simulink model "hexapod"  (R2015a)
settings: Solver=ode23tb  StartTime=0.0  StopTime=10  FixedStep=0.001  MaxStep=0.01  RelTol=1e-4  AbsTol=1e-5
values from neighbouring files (symbols this model uses):
  bL = 18.5    [runFirst.m]    (also in runFirst2.m = 20.5)
  bWb = 12.5    [runFirst.m]    (also in runFirst2.m = 14.5)
  bWs = 10.5    [runFirst.m]    (also in runFirst2.m = 12.5)
  C = CM + CL/n^2    (= 0.0001377500155)    [runFirst.m]
  d1 = 0    [runFirst.m]    (also in runFirst2.m)
  d2 = -4.61    [runFirst.m]    (also in runFirst2.m = 0)
  J = JM + JL/n^2    (= 0.008455500031)    [runFirst.m]
  Ka = 12    [runFirst.m]
  Kb = 0.00867    [runFirst.m]
  Ke = 1    [runFirst.m]
  Km = 4.375    [runFirst.m]
  L = 0.0006    [runFirst.m]
  L1 = 3.64    [runFirst.m]    (also in runFirst2.m = 3.4)
  l1x = 15.78    [runFirst.m]
  l1y = 11.78    [runFirst.m]
  l1z = -14.9    [runFirst.m]
  L2 = 5.72    [runFirst.m]    (also in runFirst2.m = 8.7)
  l2x = 0    [runFirst.m]
  l2y = 15.48    [runFirst.m]
  l2z = -14.9    [runFirst.m]
  L3 = 12.46    [runFirst.m]    (also in runFirst2.m = 12.73)
  l3x = -15.78    [runFirst.m]
  l3y = 11.78    [runFirst.m]
  l3z = -14.9    [runFirst.m]
  l4x = 15.78    [runFirst.m]
  l4y = -11.78    [runFirst.m]
  l4z = -14.9    [runFirst.m]
  l5x = 0    [runFirst.m]
  l5y = -15.48    [runFirst.m]
  l5z = -14.9    [runFirst.m]
  l6x = -15.78    [runFirst.m]
  l6y = -11.78    [runFirst.m]
  l6z = -14.9    [runFirst.m]
  n = 254    [runFirst.m]
  R = 1.4    [runFirst.m]
  stX = 4    [runFirst.m]
  stZ = 2    [runFirst.m]
  Ts = 2    [runFirst.m]
undefined symbols (not defined in the file or in its folder): X, Y, Z
undefined symbols (not defined in the file): bH, bM, m1, m2, m3
libraries: sm_lib x108, nesl_utility x52, simulink x12, Contact_Forces_Lib x7, roblocks x2
(part 2 of 5)

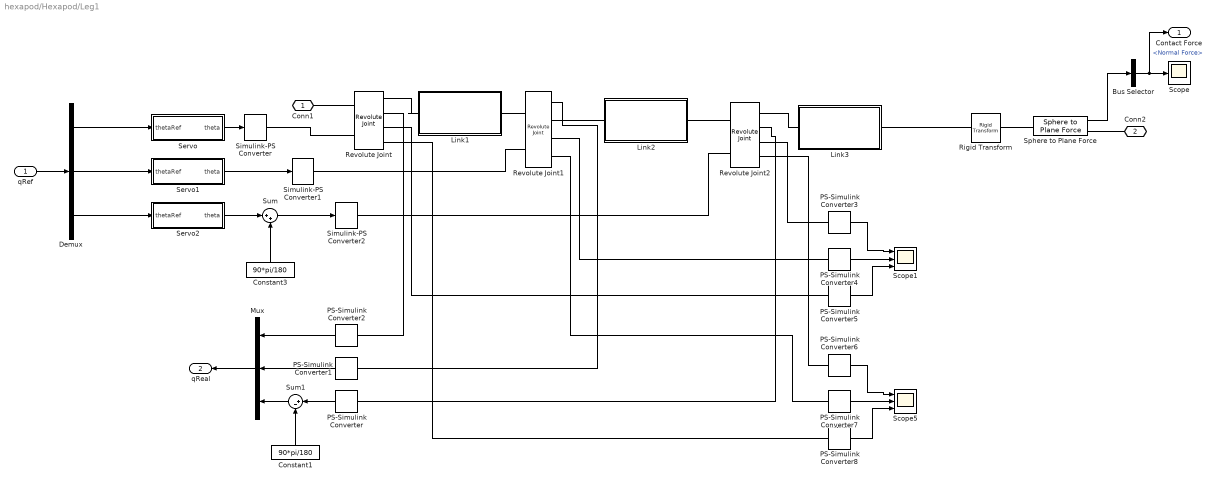
== system hexapod/Hexapod/Leg1 ==
  qRef : Inport
  Bus Selector : BusSelector  OutputSignals=Normal Force
  Constant1 : Constant  Value=90*pi/180
  Constant3 : Constant  Value=90*pi/180
  Demux : Demux  Outputs=3
  Link1 : Subsystem  mask{L=L1, W=1, H=1, m=m1, rgb=[0.1 0.1 0.90], Xangle=90, d1=-2.3}
      mask prompts: L "Length (cm)"; W "Width (cm)"; H "Thickness (cm)"; m "Mass (kg)"; rgb "Color [R G B]"; Xangle "+X Rotation (deg)"
      mask Display:
      | text(5,10, 'Link')
      | image(imread('sm_smpl_body.png'))
      | port_label('LConn',1,'L')
      | port_label('RConn',1,'R')
  Link2 : Subsystem  mask{L=L2, W=1, H=1, m=m2, rgb=[0.1 0.9 0.1], Xangle=180}
      mask prompts: L "Length (cm)"; W "Width (cm)"; H "Thickness (cm)"; m "Mass (kg)"; rgb "Color [R G B]"; Xangle "+X Rotation (deg)"
      mask Display:
      | text(5,10, 'Link')
      | image(imread('sm_smpl_body.png'))
      | port_label('LConn',1,'L')
      | port_label('RConn',1,'R')
  Link3 : Subsystem  mask{L=L3, W=1, H=1, m=m3, rgb=[0.9 0.1 0.10], Xangle=0}
      mask prompts: L "Length (cm)"; W "Width (cm)"; H "Thickness (cm)"; m "Mass (kg)"; rgb "Color [R G B]"; Xangle "+X Rotation (deg)"
      mask Display:
      | text(5,10, 'Link')
      | image(imread('sm_smpl_body.png'))
      | port_label('LConn',1,'L')
      | port_label('RConn',1,'R')
  Mux : Mux  Inputs=3
  PS-Simulink Converter{,1..8} (9 alike) : nesl_utility/PS-Simulink Converter  PhysicalDomain=network_engine_domain  SubClassName=ps_output  LeftPortType=input  RightPortType=output  PseudoPeriodic=off  Frequencies=[]  Unit=1  AffineConversion=off
  Revolute Joint : sm_lib/Joints/Revolute Joint  SenseConstraintForce=off  SenseConstraintForceX=off  SenseConstraintForceY=off  SenseConstraintForceZ=off  SenseConstraintTorque=off  SenseConstraintTorqueX=off  SenseConstraintTorqueY=off  SenseConstraintTorqueZ=off  SenseTotalForce=off  SenseTotalForceX=off  SenseTotalForceY=off  SenseTotalForceZ=off  SenseTotalTorque=on  SenseTotalTorqueX=off  SenseTotalTorqueY=off  SenseTotalTorqueZ=off  CompositeWrenchDir=FollowerOnBase  CompositeWrenchFrame=BaseFrame  EquilibriumPosition=0  EquilibriumPositionUnits=deg  SpringStiffness=0  SpringStiffnessUnits=N*m/deg  DampingCoefficient=0  DampingCoefficientUnits=N*m/(deg/s)  TorqueActuationMode=ComputedTorque  MotionActuationMode=InputMotion  SensePosition=on  SenseVelocity=off  SenseAcceleration=off  SenseTorqueForce=on  PositionTargetSpecify=off  PositionTargetPriority=High  PositionTargetValue=0  PositionTargetValueUnits=deg  VelocityTargetSpecify=off  VelocityTargetPriority=High  VelocityTargetValue=0  VelocityTargetValueUnits=deg/s  BlockFunction=simmechanics.library.joints.revolute_joint
  Revolute Joint1 : sm_lib/Joints/Revolute Joint  SenseConstraintForce=off  SenseConstraintForceX=off  SenseConstraintForceY=off  SenseConstraintForceZ=off  SenseConstraintTorque=off  SenseConstraintTorqueX=off  SenseConstraintTorqueY=off  SenseConstraintTorqueZ=off  SenseTotalForce=off  SenseTotalForceX=off  SenseTotalForceY=off  SenseTotalForceZ=off  SenseTotalTorque=on  SenseTotalTorqueX=off  SenseTotalTorqueY=off  SenseTotalTorqueZ=off  CompositeWrenchDir=FollowerOnBase  CompositeWrenchFrame=BaseFrame  EquilibriumPosition=0  EquilibriumPositionUnits=deg  SpringStiffness=0  SpringStiffnessUnits=N*m/deg  DampingCoefficient=0  DampingCoefficientUnits=N*m/(deg/s)  TorqueActuationMode=ComputedTorque  MotionActuationMode=InputMotion  SensePosition=on  SenseVelocity=off  SenseAcceleration=off  SenseTorqueForce=on  PositionTargetSpecify=off  PositionTargetPriority=High  PositionTargetValue=0  PositionTargetValueUnits=deg  VelocityTargetSpecify=off  VelocityTargetPriority=High  VelocityTargetValue=0  VelocityTargetValueUnits=deg/s  BlockFunction=simmechanics.library.joints.revolute_joint
  Revolute Joint2 : sm_lib/Joints/Revolute Joint  SenseConstraintForce=off  SenseConstraintForceX=off  SenseConstraintForceY=off  SenseConstraintForceZ=off  SenseConstraintTorque=off  SenseConstraintTorqueX=off  SenseConstraintTorqueY=off  SenseConstraintTorqueZ=off  SenseTotalForce=off  SenseTotalForceX=off  SenseTotalForceY=off  SenseTotalForceZ=off  SenseTotalTorque=on  SenseTotalTorqueX=off  SenseTotalTorqueY=off  SenseTotalTorqueZ=off  CompositeWrenchDir=FollowerOnBase  CompositeWrenchFrame=BaseFrame  EquilibriumPosition=0  EquilibriumPositionUnits=deg  SpringStiffness=0  SpringStiffnessUnits=N*m/deg  DampingCoefficient=0  DampingCoefficientUnits=N*m/(deg/s)  TorqueActuationMode=ComputedTorque  MotionActuationMode=InputMotion  SensePosition=on  SenseVelocity=off  SenseAcceleration=off  SenseTorqueForce=on  PositionTargetSpecify=off  PositionTargetPriority=High  PositionTargetValue=0  PositionTargetValueUnits=deg  VelocityTargetSpecify=off  VelocityTargetPriority=High  VelocityTargetValue=0  VelocityTargetValueUnits=deg/s  BlockFunction=simmechanics.library.joints.revolute_joint
  Rigid Transform : sm_lib/Frames and Transforms/Rigid Transform  TranslationMethod=StandardAxis  TranslationLengthUnit=m  TranslationStandardAxis=-X  TranslationStandardOffset=0.01  TranslationCartesianOffset=[0 0 0]  TranslationROffset=0  TranslationROffsetUnits=m  TranslationZOffset=0  TranslationZOffsetUnits=m  TranslationThetaOffset=0  TranslationThetaOffsetUnits=deg  RotationMethod=None  RotationAngleUnits=deg  RotationStandardAxis=+Z  RotationAngle=0.0  RotationArbitraryAxis=[0 0 1]  FollAlignAxisA=+X  BaseAlignAxisA=+Y  FollAlignAxisB=+Y  BaseAlignAxisB=+Z  RotationMatrix=[1 0 0; 0 1 0; 0 0 1]  BlockFunction=simmechanics.library.frames_transforms.rigid_transform
  Scope : Scope
      settings: YMin=0  YMax=14000  SaveName=ScopeData7
  Scope1 : Scope  NumInputPorts=3
      settings: YMin=-15~-5~-5  YMax=20~5~5  SaveName=ScopeData31
  Scope5 : Scope  NumInputPorts=3
      settings: YMin=-15~-5~-5  YMax=20~5~5  SaveName=ScopeData30
  Servo : Subsystem
  Servo1 : Subsystem
  Servo2 : Subsystem
  Simulink-PS Converter : nesl_utility/Simulink-PS Converter  PhysicalDomain=network_engine_domain  SubClassName=ps_input  LeftPortType=input  RightPortType=output  PseudoPeriodic=off  Frequencies=[]  NoiseDistribution=none  NoiseParameters=[]  Unit=1  AffineConversion=off  InputFiltering=on  SimscapeFilterOrder=2  InputFilterTimeConstant=0.001  UdotUserProvided=1
  Simulink-PS Converter1 : nesl_utility/Simulink-PS Converter  PhysicalDomain=network_engine_domain  SubClassName=ps_input  LeftPortType=input  RightPortType=output  PseudoPeriodic=off  Frequencies=[]  NoiseDistribution=none  NoiseParameters=[]  Unit=1  AffineConversion=off  InputFiltering=on  SimscapeFilterOrder=2  InputFilterTimeConstant=0.001  UdotUserProvided=1
  Simulink-PS Converter2 : nesl_utility/Simulink-PS Converter  PhysicalDomain=network_engine_domain  SubClassName=ps_input  LeftPortType=input  RightPortType=output  PseudoPeriodic=off  Frequencies=[]  NoiseDistribution=none  NoiseParameters=[]  Unit=1  AffineConversion=off  InputFiltering=on  SimscapeFilterOrder=2  InputFilterTimeConstant=0.001  UdotUserProvided=1
  Sphere to Plane Force : Contact_Forces_Lib/3D/Sphere to Plane Force  sphere_rad=0.01  plane_lenx=surfX  plane_leny=surfY  plane_depth=0.01/2  force_law=Linear  k_contact=23.9e3  b_contact=459  pen_full_damp_F=1e-4  pen_exponent=1  custom_param_1=1  custom_param_2=1  friction_law=Stick-Slip Continuous  mu_kinetic=2  mu_static=2  v_thr=0.001
  Sum : Sum  Inputs=|++
  Sum1 : Sum  Inputs=|+-
  Conn1 : PMIOPort  Port=1  Side=Left
  Conn2 : PMIOPort  Port=2  Side=Right
  Contact Force : Outport
  qReal : Outport  Port=2
  wires:
  Demux/2 -> Servo1/1(thetaRef)
  Demux/3 -> Servo2/1(thetaRef)
  Sum/1 -> Simulink-PS Converter2/1
  Constant3/1 -> Sum/2
  Demux/1 -> Servo/1(thetaRef)
  qRef/1 -> Demux/1
  Servo/1(theta) -> Simulink-PS Converter/1
  Servo1/1(theta) -> Simulink-PS Converter1/1
  Servo2/1(theta) -> Sum/1
  Sphere to Plane Force/1 -> Bus Selector/1
  Bus Selector/1 -> Contact Force/1, Scope/1  "<Normal Force>"
  Mux/1 -> qReal/1
  PS-Simulink Converter2/1 -> Mux/1
  PS-Simulink Converter1/1 -> Mux/2
  PS-Simulink Converter/1 -> Sum1/1
  Sum1/1 -> Mux/3
  Constant1/1 -> Sum1/2
  PS-Simulink Converter3/1 -> Scope1/1
  PS-Simulink Converter5/1 -> Scope1/3
  PS-Simulink Converter4/1 -> Scope1/2
  PS-Simulink Converter6/1 -> Scope5/1
  PS-Simulink Converter8/1 -> Scope5/3
  PS-Simulink Converter7/1 -> Scope5/2
  connections:
  Link1/LConn1 -- Revolute Joint/RConn1
  Revolute Joint/LConn1 -- Conn1/RConn1
  Revolute Joint/LConn2 -- Simulink-PS Converter/RConn1
  Revolute Joint1/LConn1 -- Link1/RConn1
  Revolute Joint1/RConn1 -- Link2/LConn1
  Revolute Joint2/LConn1 -- Link2/RConn1
  Revolute Joint2/RConn1 -- Link3/LConn1
  Simulink-PS Converter1/RConn1 -- Revolute Joint1/LConn2
  Revolute Joint2/LConn2 -- Simulink-PS Converter2/RConn1
  Rigid Transform/LConn1 -- Link3/RConn1
  Sphere to Plane Force/LConn1 -- Rigid Transform/RConn1
  Conn2/RConn1 -- Sphere to Plane Force/RConn1
  PS-Simulink Converter/LConn1 -- Revolute Joint2/RConn2
  PS-Simulink Converter1/LConn1 -- Revolute Joint1/RConn2
  PS-Simulink Converter2/LConn1 -- Revolute Joint/RConn2
  PS-Simulink Converter3/LConn1 -- Revolute Joint2/RConn3
  PS-Simulink Converter4/LConn1 -- Revolute Joint1/RConn3
  PS-Simulink Converter5/LConn1 -- Revolute Joint/RConn3
  PS-Simulink Converter6/LConn1 -- Revolute Joint2/RConn4
  PS-Simulink Converter7/LConn1 -- Revolute Joint1/RConn4
  PS-Simulink Converter8/LConn1 -- Revolute Joint/RConn4

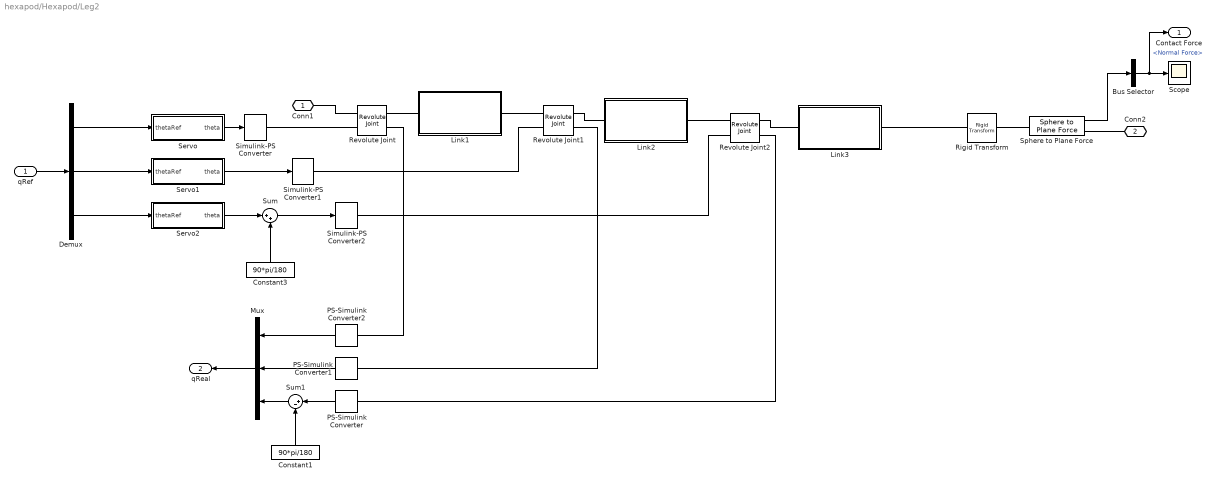
== system hexapod/Hexapod/Leg2 ==
  qRef : Inport
  Bus Selector : BusSelector  OutputSignals=Normal Force
  Constant1 : Constant  Value=90*pi/180
  Constant3 : Constant  Value=90*pi/180
  Demux : Demux  Outputs=3
  Link1 : Subsystem  mask{L=L1, W=1, H=1, m=m1, rgb=[0.1 0.1 0.90], Xangle=90}
      mask prompts: L "Length (cm)"; W "Width (cm)"; H "Thickness (cm)"; m "Mass (kg)"; rgb "Color [R G B]"; Xangle "+X Rotation (deg)"
      mask Display:
      | text(5,10, 'Link')
      | image(imread('sm_smpl_body.png'))
      | port_label('LConn',1,'L')
      | port_label('RConn',1,'R')
  Link2 : Subsystem  mask{L=L2, W=1, H=1, m=m2, rgb=[0.1 0.9 0.1], Xangle=180}
      mask prompts: L "Length (cm)"; W "Width (cm)"; H "Thickness (cm)"; m "Mass (kg)"; rgb "Color [R G B]"; Xangle "+X Rotation (deg)"
      mask Display:
      | text(5,10, 'Link')
      | image(imread('sm_smpl_body.png'))
      | port_label('LConn',1,'L')
      | port_label('RConn',1,'R')
  Link3 : Subsystem  mask{L=L3, W=1, H=1, m=m3, rgb=[0.9 0.1 0.10], Xangle=0}
      mask prompts: L "Length (cm)"; W "Width (cm)"; H "Thickness (cm)"; m "Mass (kg)"; rgb "Color [R G B]"; Xangle "+X Rotation (deg)"
      mask Display:
      | text(5,10, 'Link')
      | image(imread('sm_smpl_body.png'))
      | port_label('LConn',1,'L')
      | port_label('RConn',1,'R')
  Mux : Mux  Inputs=3
  PS-Simulink Converter : nesl_utility/PS-Simulink Converter  PhysicalDomain=network_engine_domain  SubClassName=ps_output  LeftPortType=input  RightPortType=output  PseudoPeriodic=off  Frequencies=[]  Unit=1  AffineConversion=off
  PS-Simulink Converter1 : nesl_utility/PS-Simulink Converter  PhysicalDomain=network_engine_domain  SubClassName=ps_output  LeftPortType=input  RightPortType=output  PseudoPeriodic=off  Frequencies=[]  Unit=1  AffineConversion=off
  PS-Simulink Converter2 : nesl_utility/PS-Simulink Converter  PhysicalDomain=network_engine_domain  SubClassName=ps_output  LeftPortType=input  RightPortType=output  PseudoPeriodic=off  Frequencies=[]  Unit=1  AffineConversion=off
  Revolute Joint : sm_lib/Joints/Revolute Joint  SenseConstraintForce=off  SenseConstraintForceX=off  SenseConstraintForceY=off  SenseConstraintForceZ=off  SenseConstraintTorque=off  SenseConstraintTorqueX=off  SenseConstraintTorqueY=off  SenseConstraintTorqueZ=off  SenseTotalForce=off  SenseTotalForceX=off  SenseTotalForceY=off  SenseTotalForceZ=off  SenseTotalTorque=off  SenseTotalTorqueX=off  SenseTotalTorqueY=off  SenseTotalTorqueZ=off  CompositeWrenchDir=FollowerOnBase  CompositeWrenchFrame=BaseFrame  EquilibriumPosition=0  EquilibriumPositionUnits=deg  SpringStiffness=0  SpringStiffnessUnits=N*m/deg  DampingCoefficient=0  DampingCoefficientUnits=N*m/(deg/s)  TorqueActuationMode=ComputedTorque  MotionActuationMode=InputMotion  SensePosition=on  SenseVelocity=off  SenseAcceleration=off  SenseTorqueForce=off  PositionTargetSpecify=off  PositionTargetPriority=High  PositionTargetValue=0  PositionTargetValueUnits=deg  VelocityTargetSpecify=off  VelocityTargetPriority=High  VelocityTargetValue=0  VelocityTargetValueUnits=deg/s  BlockFunction=simmechanics.library.joints.revolute_joint
  Revolute Joint1 : sm_lib/Joints/Revolute Joint  SenseConstraintForce=off  SenseConstraintForceX=off  SenseConstraintForceY=off  SenseConstraintForceZ=off  SenseConstraintTorque=off  SenseConstraintTorqueX=off  SenseConstraintTorqueY=off  SenseConstraintTorqueZ=off  SenseTotalForce=off  SenseTotalForceX=off  SenseTotalForceY=off  SenseTotalForceZ=off  SenseTotalTorque=off  SenseTotalTorqueX=off  SenseTotalTorqueY=off  SenseTotalTorqueZ=off  CompositeWrenchDir=FollowerOnBase  CompositeWrenchFrame=BaseFrame  EquilibriumPosition=0  EquilibriumPositionUnits=deg  SpringStiffness=0  SpringStiffnessUnits=N*m/deg  DampingCoefficient=0  DampingCoefficientUnits=N*m/(deg/s)  TorqueActuationMode=ComputedTorque  MotionActuationMode=InputMotion  SensePosition=on  SenseVelocity=off  SenseAcceleration=off  SenseTorqueForce=off  PositionTargetSpecify=off  PositionTargetPriority=High  PositionTargetValue=0  PositionTargetValueUnits=deg  VelocityTargetSpecify=off  VelocityTargetPriority=High  VelocityTargetValue=0  VelocityTargetValueUnits=deg/s  BlockFunction=simmechanics.library.joints.revolute_joint
  Revolute Joint2 : sm_lib/Joints/Revolute Joint  SenseConstraintForce=off  SenseConstraintForceX=off  SenseConstraintForceY=off  SenseConstraintForceZ=off  SenseConstraintTorque=off  SenseConstraintTorqueX=off  SenseConstraintTorqueY=off  SenseConstraintTorqueZ=off  SenseTotalForce=off  SenseTotalForceX=off  SenseTotalForceY=off  SenseTotalForceZ=off  SenseTotalTorque=off  SenseTotalTorqueX=off  SenseTotalTorqueY=off  SenseTotalTorqueZ=off  CompositeWrenchDir=FollowerOnBase  CompositeWrenchFrame=BaseFrame  EquilibriumPosition=0  EquilibriumPositionUnits=deg  SpringStiffness=0  SpringStiffnessUnits=N*m/deg  DampingCoefficient=0  DampingCoefficientUnits=N*m/(deg/s)  TorqueActuationMode=ComputedTorque  MotionActuationMode=InputMotion  SensePosition=on  SenseVelocity=off  SenseAcceleration=off  SenseTorqueForce=off  PositionTargetSpecify=off  PositionTargetPriority=High  PositionTargetValue=0  PositionTargetValueUnits=deg  VelocityTargetSpecify=off  VelocityTargetPriority=High  VelocityTargetValue=0  VelocityTargetValueUnits=deg/s  BlockFunction=simmechanics.library.joints.revolute_joint
  Rigid Transform : sm_lib/Frames and Transforms/Rigid Transform  TranslationMethod=StandardAxis  TranslationLengthUnit=m  TranslationStandardAxis=-X  TranslationStandardOffset=0.01  TranslationCartesianOffset=[0 0 0]  TranslationROffset=0  TranslationROffsetUnits=m  TranslationZOffset=0  TranslationZOffsetUnits=m  TranslationThetaOffset=0  TranslationThetaOffsetUnits=deg  RotationMethod=None  RotationAngleUnits=deg  RotationStandardAxis=+Z  RotationAngle=0.0  RotationArbitraryAxis=[0 0 1]  FollAlignAxisA=+X  BaseAlignAxisA=+Y  FollAlignAxisB=+Y  BaseAlignAxisB=+Z  RotationMatrix=[1 0 0; 0 1 0; 0 0 1]  BlockFunction=simmechanics.library.frames_transforms.rigid_transform
  Scope : Scope
      settings: YMin=0  YMax=14000  SaveName=ScopeData7
  Servo : Subsystem
  Servo1 : Subsystem
  Servo2 : Subsystem
  Simulink-PS Converter : nesl_utility/Simulink-PS Converter  PhysicalDomain=network_engine_domain  SubClassName=ps_input  LeftPortType=input  RightPortType=output  PseudoPeriodic=off  Frequencies=[]  NoiseDistribution=none  NoiseParameters=[]  Unit=1  AffineConversion=off  InputFiltering=on  SimscapeFilterOrder=2  InputFilterTimeConstant=0.001  UdotUserProvided=1
  Simulink-PS Converter1 : nesl_utility/Simulink-PS Converter  PhysicalDomain=network_engine_domain  SubClassName=ps_input  LeftPortType=input  RightPortType=output  PseudoPeriodic=off  Frequencies=[]  NoiseDistribution=none  NoiseParameters=[]  Unit=1  AffineConversion=off  InputFiltering=on  SimscapeFilterOrder=2  InputFilterTimeConstant=0.001  UdotUserProvided=1
  Simulink-PS Converter2 : nesl_utility/Simulink-PS Converter  PhysicalDomain=network_engine_domain  SubClassName=ps_input  LeftPortType=input  RightPortType=output  PseudoPeriodic=off  Frequencies=[]  NoiseDistribution=none  NoiseParameters=[]  Unit=1  AffineConversion=off  InputFiltering=on  SimscapeFilterOrder=2  InputFilterTimeConstant=0.001  UdotUserProvided=1
  Sphere to Plane Force : Contact_Forces_Lib/3D/Sphere to Plane Force  sphere_rad=0.01  plane_lenx=surfX  plane_leny=surfY  plane_depth=0.01/2  force_law=Linear  k_contact=23.9e3  b_contact=459  pen_full_damp_F=1e-4  pen_exponent=1  custom_param_1=1  custom_param_2=1  friction_law=Stick-Slip Continuous  mu_kinetic=2  mu_static=2  v_thr=0.001
  Sum : Sum  Inputs=|++
  Sum1 : Sum  Inputs=|+-
  Conn1 : PMIOPort  Port=1  Side=Left
  Conn2 : PMIOPort  Port=2  Side=Right
  Contact Force : Outport
  qReal : Outport  Port=2
  wires:
  Constant1/1 -> Sum1/2
  Sum1/1 -> Mux/3
  PS-Simulink Converter/1 -> Sum1/1
  PS-Simulink Converter1/1 -> Mux/2
  PS-Simulink Converter2/1 -> Mux/1
  Mux/1 -> qReal/1
  Bus Selector/1 -> Scope/1, Contact Force/1  "<Normal Force>"
  Sphere to Plane Force/1 -> Bus Selector/1
  Servo2/1(theta) -> Sum/1
  Servo1/1(theta) -> Simulink-PS Converter1/1
  Servo/1(theta) -> Simulink-PS Converter/1
  qRef/1 -> Demux/1
  Demux/1 -> Servo/1(thetaRef)
  Constant3/1 -> Sum/2
  Sum/1 -> Simulink-PS Converter2/1
  Demux/3 -> Servo2/1(thetaRef)
  Demux/2 -> Servo1/1(thetaRef)
  connections:
  PS-Simulink Converter2/LConn1 -- Revolute Joint/RConn2
  PS-Simulink Converter1/LConn1 -- Revolute Joint1/RConn2
  PS-Simulink Converter/LConn1 -- Revolute Joint2/RConn2
  Sphere to Plane Force/RConn1 -- Conn2/RConn1
  Rigid Transform/LConn1 -- Link3/RConn1
  Revolute Joint2/LConn2 -- Simulink-PS Converter2/RConn1
  Simulink-PS Converter1/RConn1 -- Revolute Joint1/LConn2
  Revolute Joint2/RConn1 -- Link3/LConn1
  Revolute Joint2/LConn1 -- Link2/RConn1
  Revolute Joint1/RConn1 -- Link2/LConn1
  Revolute Joint1/LConn1 -- Link1/RConn1
  Revolute Joint/LConn2 -- Simulink-PS Converter/RConn1
  Revolute Joint/LConn1 -- Conn1/RConn1
  Link1/LConn1 -- Revolute Joint/RConn1
  Sphere to Plane Force/LConn1 -- Rigid Transform/RConn1

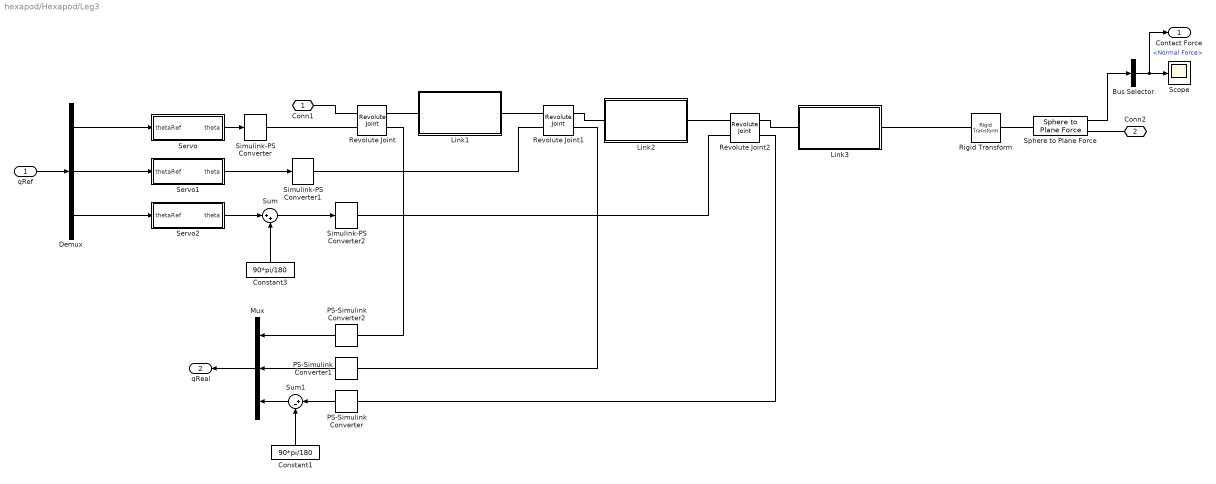
== system hexapod/Hexapod/Leg3 ==
  qRef : Inport
  Bus Selector : BusSelector  OutputSignals=Normal Force
  Constant1 : Constant  Value=90*pi/180
  Constant3 : Constant  Value=90*pi/180
  Demux : Demux  Outputs=3
  Link1 : Subsystem  mask{L=L1, W=1, H=1, m=m1, rgb=[0.1 0.1 0.90], Xangle=90}
      mask prompts: L "Length (cm)"; W "Width (cm)"; H "Thickness (cm)"; m "Mass (kg)"; rgb "Color [R G B]"; Xangle "+X Rotation (deg)"
      mask Display:
      | text(5,10, 'Link')
      | image(imread('sm_smpl_body.png'))
      | port_label('LConn',1,'L')
      | port_label('RConn',1,'R')
  Link2 : Subsystem  mask{L=L2, W=1, H=1, m=m2, rgb=[0.1 0.9 0.1], Xangle=180}
      mask prompts: L "Length (cm)"; W "Width (cm)"; H "Thickness (cm)"; m "Mass (kg)"; rgb "Color [R G B]"; Xangle "+X Rotation (deg)"
      mask Display:
      | text(5,10, 'Link')
      | image(imread('sm_smpl_body.png'))
      | port_label('LConn',1,'L')
      | port_label('RConn',1,'R')
  Link3 : Subsystem  mask{L=L3, W=1, H=1, m=m3, rgb=[0.9 0.1 0.10], Xangle=0}
      mask prompts: L "Length (cm)"; W "Width (cm)"; H "Thickness (cm)"; m "Mass (kg)"; rgb "Color [R G B]"; Xangle "+X Rotation (deg)"
      mask Display:
      | text(5,10, 'Link')
      | image(imread('sm_smpl_body.png'))
      | port_label('LConn',1,'L')
      | port_label('RConn',1,'R')
  Mux : Mux  Inputs=3
  PS-Simulink Converter : nesl_utility/PS-Simulink Converter  PhysicalDomain=network_engine_domain  SubClassName=ps_output  LeftPortType=input  RightPortType=output  PseudoPeriodic=off  Frequencies=[]  Unit=1  AffineConversion=off
  PS-Simulink Converter1 : nesl_utility/PS-Simulink Converter  PhysicalDomain=network_engine_domain  SubClassName=ps_output  LeftPortType=input  RightPortType=output  PseudoPeriodic=off  Frequencies=[]  Unit=1  AffineConversion=off
  PS-Simulink Converter2 : nesl_utility/PS-Simulink Converter  PhysicalDomain=network_engine_domain  SubClassName=ps_output  LeftPortType=input  RightPortType=output  PseudoPeriodic=off  Frequencies=[]  Unit=1  AffineConversion=off
  Revolute Joint : sm_lib/Joints/Revolute Joint  SenseConstraintForce=off  SenseConstraintForceX=off  SenseConstraintForceY=off  SenseConstraintForceZ=off  SenseConstraintTorque=off  SenseConstraintTorqueX=off  SenseConstraintTorqueY=off  SenseConstraintTorqueZ=off  SenseTotalForce=off  SenseTotalForceX=off  SenseTotalForceY=off  SenseTotalForceZ=off  SenseTotalTorque=off  SenseTotalTorqueX=off  SenseTotalTorqueY=off  SenseTotalTorqueZ=off  CompositeWrenchDir=FollowerOnBase  CompositeWrenchFrame=BaseFrame  EquilibriumPosition=0  EquilibriumPositionUnits=deg  SpringStiffness=0  SpringStiffnessUnits=N*m/deg  DampingCoefficient=0  DampingCoefficientUnits=N*m/(deg/s)  TorqueActuationMode=ComputedTorque  MotionActuationMode=InputMotion  SensePosition=on  SenseVelocity=off  SenseAcceleration=off  SenseTorqueForce=off  PositionTargetSpecify=off  PositionTargetPriority=High  PositionTargetValue=0  PositionTargetValueUnits=deg  VelocityTargetSpecify=off  VelocityTargetPriority=High  VelocityTargetValue=0  VelocityTargetValueUnits=deg/s  BlockFunction=simmechanics.library.joints.revolute_joint
  Revolute Joint1 : sm_lib/Joints/Revolute Joint  SenseConstraintForce=off  SenseConstraintForceX=off  SenseConstraintForceY=off  SenseConstraintForceZ=off  SenseConstraintTorque=off  SenseConstraintTorqueX=off  SenseConstraintTorqueY=off  SenseConstraintTorqueZ=off  SenseTotalForce=off  SenseTotalForceX=off  SenseTotalForceY=off  SenseTotalForceZ=off  SenseTotalTorque=off  SenseTotalTorqueX=off  SenseTotalTorqueY=off  SenseTotalTorqueZ=off  CompositeWrenchDir=FollowerOnBase  CompositeWrenchFrame=BaseFrame  EquilibriumPosition=0  EquilibriumPositionUnits=deg  SpringStiffness=0  SpringStiffnessUnits=N*m/deg  DampingCoefficient=0  DampingCoefficientUnits=N*m/(deg/s)  TorqueActuationMode=ComputedTorque  MotionActuationMode=InputMotion  SensePosition=on  SenseVelocity=off  SenseAcceleration=off  SenseTorqueForce=off  PositionTargetSpecify=off  PositionTargetPriority=High  PositionTargetValue=0  PositionTargetValueUnits=deg  VelocityTargetSpecify=off  VelocityTargetPriority=High  VelocityTargetValue=0  VelocityTargetValueUnits=deg/s  BlockFunction=simmechanics.library.joints.revolute_joint
  Revolute Joint2 : sm_lib/Joints/Revolute Joint  SenseConstraintForce=off  SenseConstraintForceX=off  SenseConstraintForceY=off  SenseConstraintForceZ=off  SenseConstraintTorque=off  SenseConstraintTorqueX=off  SenseConstraintTorqueY=off  SenseConstraintTorqueZ=off  SenseTotalForce=off  SenseTotalForceX=off  SenseTotalForceY=off  SenseTotalForceZ=off  SenseTotalTorque=off  SenseTotalTorqueX=off  SenseTotalTorqueY=off  SenseTotalTorqueZ=off  CompositeWrenchDir=FollowerOnBase  CompositeWrenchFrame=BaseFrame  EquilibriumPosition=0  EquilibriumPositionUnits=deg  SpringStiffness=0  SpringStiffnessUnits=N*m/deg  DampingCoefficient=0  DampingCoefficientUnits=N*m/(deg/s)  TorqueActuationMode=ComputedTorque  MotionActuationMode=InputMotion  SensePosition=on  SenseVelocity=off  SenseAcceleration=off  SenseTorqueForce=off  PositionTargetSpecify=off  PositionTargetPriority=High  PositionTargetValue=0  PositionTargetValueUnits=deg  VelocityTargetSpecify=off  VelocityTargetPriority=High  VelocityTargetValue=0  VelocityTargetValueUnits=deg/s  BlockFunction=simmechanics.library.joints.revolute_joint
  Rigid Transform : sm_lib/Frames and Transforms/Rigid Transform  TranslationMethod=StandardAxis  TranslationLengthUnit=m  TranslationStandardAxis=-X  TranslationStandardOffset=0.01  TranslationCartesianOffset=[0 0 0]  TranslationROffset=0  TranslationROffsetUnits=m  TranslationZOffset=0  TranslationZOffsetUnits=m  TranslationThetaOffset=0  TranslationThetaOffsetUnits=deg  RotationMethod=None  RotationAngleUnits=deg  RotationStandardAxis=+Z  RotationAngle=0.0  RotationArbitraryAxis=[0 0 1]  FollAlignAxisA=+X  BaseAlignAxisA=+Y  FollAlignAxisB=+Y  BaseAlignAxisB=+Z  RotationMatrix=[1 0 0; 0 1 0; 0 0 1]  BlockFunction=simmechanics.library.frames_transforms.rigid_transform
  Scope : Scope
      settings: YMin=0  YMax=14000  SaveName=ScopeData7
  Servo : Subsystem
  Servo1 : Subsystem
  Servo2 : Subsystem
  Simulink-PS Converter : nesl_utility/Simulink-PS Converter  PhysicalDomain=network_engine_domain  SubClassName=ps_input  LeftPortType=input  RightPortType=output  PseudoPeriodic=off  Frequencies=[]  NoiseDistribution=none  NoiseParameters=[]  Unit=1  AffineConversion=off  InputFiltering=on  SimscapeFilterOrder=2  InputFilterTimeConstant=0.001  UdotUserProvided=1
  Simulink-PS Converter1 : nesl_utility/Simulink-PS Converter  PhysicalDomain=network_engine_domain  SubClassName=ps_input  LeftPortType=input  RightPortType=output  PseudoPeriodic=off  Frequencies=[]  NoiseDistribution=none  NoiseParameters=[]  Unit=1  AffineConversion=off  InputFiltering=on  SimscapeFilterOrder=2  InputFilterTimeConstant=0.001  UdotUserProvided=1
  Simulink-PS Converter2 : nesl_utility/Simulink-PS Converter  PhysicalDomain=network_engine_domain  SubClassName=ps_input  LeftPortType=input  RightPortType=output  PseudoPeriodic=off  Frequencies=[]  NoiseDistribution=none  NoiseParameters=[]  Unit=1  AffineConversion=off  InputFiltering=on  SimscapeFilterOrder=2  InputFilterTimeConstant=0.001  UdotUserProvided=1
  Sphere to Plane Force : Contact_Forces_Lib/3D/Sphere to Plane Force  sphere_rad=0.01  plane_lenx=surfX  plane_leny=surfY  plane_depth=0.01/2  force_law=Linear  k_contact=23.9e3  b_contact=459  pen_full_damp_F=1e-4  pen_exponent=1  custom_param_1=1  custom_param_2=1  friction_law=Stick-Slip Continuous  mu_kinetic=2  mu_static=2  v_thr=0.001
  Sum : Sum  Inputs=|++
  Sum1 : Sum  Inputs=|+-
  Conn1 : PMIOPort  Port=1  Side=Left
  Conn2 : PMIOPort  Port=2  Side=Right
  Contact Force : Outport
  qReal : Outport  Port=2
  wires:
  Demux/2 -> Servo1/1(thetaRef)
  Demux/3 -> Servo2/1(thetaRef)
  Sum/1 -> Simulink-PS Converter2/1
  Constant3/1 -> Sum/2
  Demux/1 -> Servo/1(thetaRef)
  qRef/1 -> Demux/1
  Servo/1(theta) -> Simulink-PS Converter/1
  Servo1/1(theta) -> Simulink-PS Converter1/1
  Servo2/1(theta) -> Sum/1
  Sphere to Plane Force/1 -> Bus Selector/1
  Bus Selector/1 -> Contact Force/1, Scope/1  "<Normal Force>"
  Mux/1 -> qReal/1
  PS-Simulink Converter2/1 -> Mux/1
  PS-Simulink Converter1/1 -> Mux/2
  PS-Simulink Converter/1 -> Sum1/1
  Sum1/1 -> Mux/3
  Constant1/1 -> Sum1/2
  connections:
  Link1/LConn1 -- Revolute Joint/RConn1
  Revolute Joint/LConn1 -- Conn1/RConn1
  Revolute Joint/LConn2 -- Simulink-PS Converter/RConn1
  Revolute Joint1/LConn1 -- Link1/RConn1
  Revolute Joint1/RConn1 -- Link2/LConn1
  Revolute Joint2/LConn1 -- Link2/RConn1
  Revolute Joint2/RConn1 -- Link3/LConn1
  Simulink-PS Converter1/RConn1 -- Revolute Joint1/LConn2
  Revolute Joint2/LConn2 -- Simulink-PS Converter2/RConn1
  Rigid Transform/LConn1 -- Link3/RConn1
  Sphere to Plane Force/RConn1 -- Conn2/RConn1
  PS-Simulink Converter/LConn1 -- Revolute Joint2/RConn2
  PS-Simulink Converter1/LConn1 -- Revolute Joint1/RConn2
  PS-Simulink Converter2/LConn1 -- Revolute Joint/RConn2
  Sphere to Plane Force/LConn1 -- Rigid Transform/RConn1

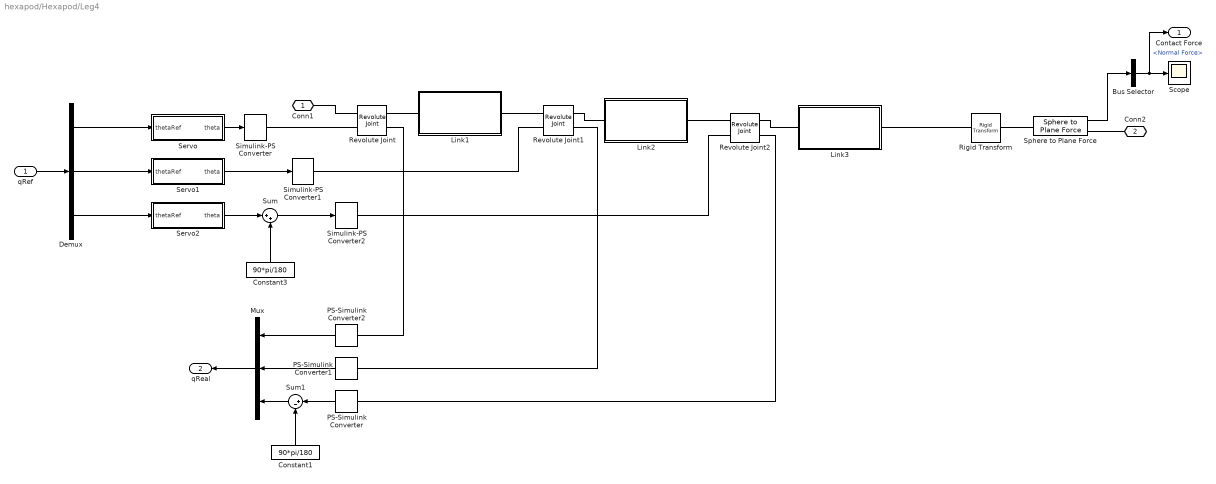
== system hexapod/Hexapod/Leg4 ==
  qRef : Inport
  Bus Selector : BusSelector  OutputSignals=Normal Force
  Constant1 : Constant  Value=90*pi/180
  Constant3 : Constant  Value=90*pi/180
  Demux : Demux  Outputs=3
  Link1 : Subsystem  mask{L=L1, W=1, H=1, m=m1, rgb=[0.1 0.1 0.90], Xangle=90}
      mask prompts: L "Length (cm)"; W "Width (cm)"; H "Thickness (cm)"; m "Mass (kg)"; rgb "Color [R G B]"; Xangle "+X Rotation (deg)"
      mask Display:
      | text(5,10, 'Link')
      | image(imread('sm_smpl_body.png'))
      | port_label('LConn',1,'L')
      | port_label('RConn',1,'R')
  Link2 : Subsystem  mask{L=L2, W=1, H=1, m=m2, rgb=[0.1 0.9 0.1], Xangle=180}
      mask prompts: L "Length (cm)"; W "Width (cm)"; H "Thickness (cm)"; m "Mass (kg)"; rgb "Color [R G B]"; Xangle "+X Rotation (deg)"
      mask Display:
      | text(5,10, 'Link')
      | image(imread('sm_smpl_body.png'))
      | port_label('LConn',1,'L')
      | port_label('RConn',1,'R')
  Link3 : Subsystem  mask{L=L3, W=1, H=1, m=m3, rgb=[0.9 0.1 0.10], Xangle=0}
      mask prompts: L "Length (cm)"; W "Width (cm)"; H "Thickness (cm)"; m "Mass (kg)"; rgb "Color [R G B]"; Xangle "+X Rotation (deg)"
      mask Display:
      | text(5,10, 'Link')
      | image(imread('sm_smpl_body.png'))
      | port_label('LConn',1,'L')
      | port_label('RConn',1,'R')
  Mux : Mux  Inputs=3
  PS-Simulink Converter : nesl_utility/PS-Simulink Converter  PhysicalDomain=network_engine_domain  SubClassName=ps_output  LeftPortType=input  RightPortType=output  PseudoPeriodic=off  Frequencies=[]  Unit=1  AffineConversion=off
  PS-Simulink Converter1 : nesl_utility/PS-Simulink Converter  PhysicalDomain=network_engine_domain  SubClassName=ps_output  LeftPortType=input  RightPortType=output  PseudoPeriodic=off  Frequencies=[]  Unit=1  AffineConversion=off
  PS-Simulink Converter2 : nesl_utility/PS-Simulink Converter  PhysicalDomain=network_engine_domain  SubClassName=ps_output  LeftPortType=input  RightPortType=output  PseudoPeriodic=off  Frequencies=[]  Unit=1  AffineConversion=off
  Revolute Joint : sm_lib/Joints/Revolute Joint  SenseConstraintForce=off  SenseConstraintForceX=off  SenseConstraintForceY=off  SenseConstraintForceZ=off  SenseConstraintTorque=off  SenseConstraintTorqueX=off  SenseConstraintTorqueY=off  SenseConstraintTorqueZ=off  SenseTotalForce=off  SenseTotalForceX=off  SenseTotalForceY=off  SenseTotalForceZ=off  SenseTotalTorque=off  SenseTotalTorqueX=off  SenseTotalTorqueY=off  SenseTotalTorqueZ=off  CompositeWrenchDir=FollowerOnBase  CompositeWrenchFrame=BaseFrame  EquilibriumPosition=0  EquilibriumPositionUnits=deg  SpringStiffness=0  SpringStiffnessUnits=N*m/deg  DampingCoefficient=0  DampingCoefficientUnits=N*m/(deg/s)  TorqueActuationMode=ComputedTorque  MotionActuationMode=InputMotion  SensePosition=on  SenseVelocity=off  SenseAcceleration=off  SenseTorqueForce=off  PositionTargetSpecify=off  PositionTargetPriority=High  PositionTargetValue=0  PositionTargetValueUnits=deg  VelocityTargetSpecify=off  VelocityTargetPriority=High  VelocityTargetValue=0  VelocityTargetValueUnits=deg/s  BlockFunction=simmechanics.library.joints.revolute_joint
  Revolute Joint1 : sm_lib/Joints/Revolute Joint  SenseConstraintForce=off  SenseConstraintForceX=off  SenseConstraintForceY=off  SenseConstraintForceZ=off  SenseConstraintTorque=off  SenseConstraintTorqueX=off  SenseConstraintTorqueY=off  SenseConstraintTorqueZ=off  SenseTotalForce=off  SenseTotalForceX=off  SenseTotalForceY=off  SenseTotalForceZ=off  SenseTotalTorque=off  SenseTotalTorqueX=off  SenseTotalTorqueY=off  SenseTotalTorqueZ=off  CompositeWrenchDir=FollowerOnBase  CompositeWrenchFrame=BaseFrame  EquilibriumPosition=0  EquilibriumPositionUnits=deg  SpringStiffness=0  SpringStiffnessUnits=N*m/deg  DampingCoefficient=0  DampingCoefficientUnits=N*m/(deg/s)  TorqueActuationMode=ComputedTorque  MotionActuationMode=InputMotion  SensePosition=on  SenseVelocity=off  SenseAcceleration=off  SenseTorqueForce=off  PositionTargetSpecify=off  PositionTargetPriority=High  PositionTargetValue=0  PositionTargetValueUnits=deg  VelocityTargetSpecify=off  VelocityTargetPriority=High  VelocityTargetValue=0  VelocityTargetValueUnits=deg/s  BlockFunction=simmechanics.library.joints.revolute_joint
  Revolute Joint2 : sm_lib/Joints/Revolute Joint  SenseConstraintForce=off  SenseConstraintForceX=off  SenseConstraintForceY=off  SenseConstraintForceZ=off  SenseConstraintTorque=off  SenseConstraintTorqueX=off  SenseConstraintTorqueY=off  SenseConstraintTorqueZ=off  SenseTotalForce=off  SenseTotalForceX=off  SenseTotalForceY=off  SenseTotalForceZ=off  SenseTotalTorque=off  SenseTotalTorqueX=off  SenseTotalTorqueY=off  SenseTotalTorqueZ=off  CompositeWrenchDir=FollowerOnBase  CompositeWrenchFrame=BaseFrame  EquilibriumPosition=0  EquilibriumPositionUnits=deg  SpringStiffness=0  SpringStiffnessUnits=N*m/deg  DampingCoefficient=0  DampingCoefficientUnits=N*m/(deg/s)  TorqueActuationMode=ComputedTorque  MotionActuationMode=InputMotion  SensePosition=on  SenseVelocity=off  SenseAcceleration=off  SenseTorqueForce=off  PositionTargetSpecify=off  PositionTargetPriority=High  PositionTargetValue=0  PositionTargetValueUnits=deg  VelocityTargetSpecify=off  VelocityTargetPriority=High  VelocityTargetValue=0  VelocityTargetValueUnits=deg/s  BlockFunction=simmechanics.library.joints.revolute_joint
  Rigid Transform : sm_lib/Frames and Transforms/Rigid Transform  TranslationMethod=StandardAxis  TranslationLengthUnit=m  TranslationStandardAxis=-X  TranslationStandardOffset=0.01  TranslationCartesianOffset=[0 0 0]  TranslationROffset=0  TranslationROffsetUnits=m  TranslationZOffset=0  TranslationZOffsetUnits=m  TranslationThetaOffset=0  TranslationThetaOffsetUnits=deg  RotationMethod=None  RotationAngleUnits=deg  RotationStandardAxis=+Z  RotationAngle=0.0  RotationArbitraryAxis=[0 0 1]  FollAlignAxisA=+X  BaseAlignAxisA=+Y  FollAlignAxisB=+Y  BaseAlignAxisB=+Z  RotationMatrix=[1 0 0; 0 1 0; 0 0 1]  BlockFunction=simmechanics.library.frames_transforms.rigid_transform
  Scope : Scope
      settings: YMin=0  YMax=14000  SaveName=ScopeData7
  Servo : Subsystem
  Servo1 : Subsystem
  Servo2 : Subsystem
  Simulink-PS Converter : nesl_utility/Simulink-PS Converter  PhysicalDomain=network_engine_domain  SubClassName=ps_input  LeftPortType=input  RightPortType=output  PseudoPeriodic=off  Frequencies=[]  NoiseDistribution=none  NoiseParameters=[]  Unit=1  AffineConversion=off  InputFiltering=on  SimscapeFilterOrder=2  InputFilterTimeConstant=0.001  UdotUserProvided=1
  Simulink-PS Converter1 : nesl_utility/Simulink-PS Converter  PhysicalDomain=network_engine_domain  SubClassName=ps_input  LeftPortType=input  RightPortType=output  PseudoPeriodic=off  Frequencies=[]  NoiseDistribution=none  NoiseParameters=[]  Unit=1  AffineConversion=off  InputFiltering=on  SimscapeFilterOrder=2  InputFilterTimeConstant=0.001  UdotUserProvided=1
  Simulink-PS Converter2 : nesl_utility/Simulink-PS Converter  PhysicalDomain=network_engine_domain  SubClassName=ps_input  LeftPortType=input  RightPortType=output  PseudoPeriodic=off  Frequencies=[]  NoiseDistribution=none  NoiseParameters=[]  Unit=1  AffineConversion=off  InputFiltering=on  SimscapeFilterOrder=2  InputFilterTimeConstant=0.001  UdotUserProvided=1
  Sphere to Plane Force : Contact_Forces_Lib/3D/Sphere to Plane Force  sphere_rad=0.01  plane_lenx=surfX  plane_leny=surfY  plane_depth=0.01/2  force_law=Linear  k_contact=23.9e3  b_contact=459  pen_full_damp_F=1e-4  pen_exponent=1  custom_param_1=1  custom_param_2=1  friction_law=Stick-Slip Continuous  mu_kinetic=2  mu_static=2  v_thr=0.001
  Sum : Sum  Inputs=|++
  Sum1 : Sum  Inputs=|+-
  Conn1 : PMIOPort  Port=1  Side=Left
  Conn2 : PMIOPort  Port=2  Side=Right
  Contact Force : Outport
  qReal : Outport  Port=2
  wires:
  Constant1/1 -> Sum1/2
  Sum1/1 -> Mux/3
  PS-Simulink Converter/1 -> Sum1/1
  PS-Simulink Converter1/1 -> Mux/2
  PS-Simulink Converter2/1 -> Mux/1
  Mux/1 -> qReal/1
  Bus Selector/1 -> Scope/1, Contact Force/1  "<Normal Force>"
  Sphere to Plane Force/1 -> Bus Selector/1
  Servo2/1(theta) -> Sum/1
  Servo1/1(theta) -> Simulink-PS Converter1/1
  Servo/1(theta) -> Simulink-PS Converter/1
  qRef/1 -> Demux/1
  Demux/1 -> Servo/1(thetaRef)
  Constant3/1 -> Sum/2
  Sum/1 -> Simulink-PS Converter2/1
  Demux/3 -> Servo2/1(thetaRef)
  Demux/2 -> Servo1/1(thetaRef)
  connections:
  PS-Simulink Converter2/LConn1 -- Revolute Joint/RConn2
  PS-Simulink Converter1/LConn1 -- Revolute Joint1/RConn2
  PS-Simulink Converter/LConn1 -- Revolute Joint2/RConn2
  Sphere to Plane Force/RConn1 -- Conn2/RConn1
  Rigid Transform/LConn1 -- Link3/RConn1
  Revolute Joint2/LConn2 -- Simulink-PS Converter2/RConn1
  Simulink-PS Converter1/RConn1 -- Revolute Joint1/LConn2
  Revolute Joint2/RConn1 -- Link3/LConn1
  Revolute Joint2/LConn1 -- Link2/RConn1
  Revolute Joint1/RConn1 -- Link2/LConn1
  Revolute Joint1/LConn1 -- Link1/RConn1
  Revolute Joint/LConn2 -- Simulink-PS Converter/RConn1
  Revolute Joint/LConn1 -- Conn1/RConn1
  Link1/LConn1 -- Revolute Joint/RConn1
  Sphere to Plane Force/LConn1 -- Rigid Transform/RConn1

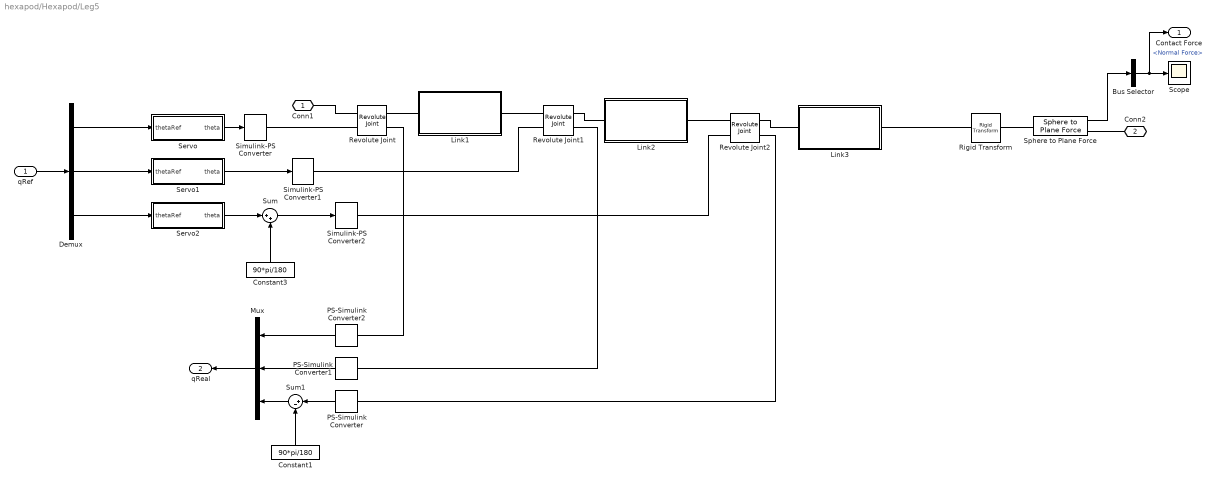
== system hexapod/Hexapod/Leg5 ==
  qRef : Inport
  Bus Selector : BusSelector  OutputSignals=Normal Force
  Constant1 : Constant  Value=90*pi/180
  Constant3 : Constant  Value=90*pi/180
  Demux : Demux  Outputs=3
  Link1 : Subsystem  mask{L=L1, W=1, H=1, m=m1, rgb=[0.1 0.1 0.90], Xangle=90}
      mask prompts: L "Length (cm)"; W "Width (cm)"; H "Thickness (cm)"; m "Mass (kg)"; rgb "Color [R G B]"; Xangle "+X Rotation (deg)"
      mask Display:
      | text(5,10, 'Link')
      | image(imread('sm_smpl_body.png'))
      | port_label('LConn',1,'L')
      | port_label('RConn',1,'R')
  Link2 : Subsystem  mask{L=L2, W=1, H=1, m=m2, rgb=[0.1 0.9 0.1], Xangle=180}
      mask prompts: L "Length (cm)"; W "Width (cm)"; H "Thickness (cm)"; m "Mass (kg)"; rgb "Color [R G B]"; Xangle "+X Rotation (deg)"
      mask Display:
      | text(5,10, 'Link')
      | image(imread('sm_smpl_body.png'))
      | port_label('LConn',1,'L')
      | port_label('RConn',1,'R')
  Link3 : Subsystem  mask{L=L3, W=1, H=1, m=m3, rgb=[0.9 0.1 0.10], Xangle=0}
      mask prompts: L "Length (cm)"; W "Width (cm)"; H "Thickness (cm)"; m "Mass (kg)"; rgb "Color [R G B]"; Xangle "+X Rotation (deg)"
      mask Display:
      | text(5,10, 'Link')
      | image(imread('sm_smpl_body.png'))
      | port_label('LConn',1,'L')
      | port_label('RConn',1,'R')
  Mux : Mux  Inputs=3
  PS-Simulink Converter : nesl_utility/PS-Simulink Converter  PhysicalDomain=network_engine_domain  SubClassName=ps_output  LeftPortType=input  RightPortType=output  PseudoPeriodic=off  Frequencies=[]  Unit=1  AffineConversion=off
  PS-Simulink Converter1 : nesl_utility/PS-Simulink Converter  PhysicalDomain=network_engine_domain  SubClassName=ps_output  LeftPortType=input  RightPortType=output  PseudoPeriodic=off  Frequencies=[]  Unit=1  AffineConversion=off
  PS-Simulink Converter2 : nesl_utility/PS-Simulink Converter  PhysicalDomain=network_engine_domain  SubClassName=ps_output  LeftPortType=input  RightPortType=output  PseudoPeriodic=off  Frequencies=[]  Unit=1  AffineConversion=off
  Revolute Joint : sm_lib/Joints/Revolute Joint  SenseConstraintForce=off  SenseConstraintForceX=off  SenseConstraintForceY=off  SenseConstraintForceZ=off  SenseConstraintTorque=off  SenseConstraintTorqueX=off  SenseConstraintTorqueY=off  SenseConstraintTorqueZ=off  SenseTotalForce=off  SenseTotalForceX=off  SenseTotalForceY=off  SenseTotalForceZ=off  SenseTotalTorque=off  SenseTotalTorqueX=off  SenseTotalTorqueY=off  SenseTotalTorqueZ=off  CompositeWrenchDir=FollowerOnBase  CompositeWrenchFrame=BaseFrame  EquilibriumPosition=0  EquilibriumPositionUnits=deg  SpringStiffness=0  SpringStiffnessUnits=N*m/deg  DampingCoefficient=0  DampingCoefficientUnits=N*m/(deg/s)  TorqueActuationMode=ComputedTorque  MotionActuationMode=InputMotion  SensePosition=on  SenseVelocity=off  SenseAcceleration=off  SenseTorqueForce=off  PositionTargetSpecify=off  PositionTargetPriority=High  PositionTargetValue=0  PositionTargetValueUnits=deg  VelocityTargetSpecify=off  VelocityTargetPriority=High  VelocityTargetValue=0  VelocityTargetValueUnits=deg/s  BlockFunction=simmechanics.library.joints.revolute_joint
  Revolute Joint1 : sm_lib/Joints/Revolute Joint  SenseConstraintForce=off  SenseConstraintForceX=off  SenseConstraintForceY=off  SenseConstraintForceZ=off  SenseConstraintTorque=off  SenseConstraintTorqueX=off  SenseConstraintTorqueY=off  SenseConstraintTorqueZ=off  SenseTotalForce=off  SenseTotalForceX=off  SenseTotalForceY=off  SenseTotalForceZ=off  SenseTotalTorque=off  SenseTotalTorqueX=off  SenseTotalTorqueY=off  SenseTotalTorqueZ=off  CompositeWrenchDir=FollowerOnBase  CompositeWrenchFrame=BaseFrame  EquilibriumPosition=0  EquilibriumPositionUnits=deg  SpringStiffness=0  SpringStiffnessUnits=N*m/deg  DampingCoefficient=0  DampingCoefficientUnits=N*m/(deg/s)  TorqueActuationMode=ComputedTorque  MotionActuationMode=InputMotion  SensePosition=on  SenseVelocity=off  SenseAcceleration=off  SenseTorqueForce=off  PositionTargetSpecify=off  PositionTargetPriority=High  PositionTargetValue=0  PositionTargetValueUnits=deg  VelocityTargetSpecify=off  VelocityTargetPriority=High  VelocityTargetValue=0  VelocityTargetValueUnits=deg/s  BlockFunction=simmechanics.library.joints.revolute_joint
  Revolute Joint2 : sm_lib/Joints/Revolute Joint  SenseConstraintForce=off  SenseConstraintForceX=off  SenseConstraintForceY=off  SenseConstraintForceZ=off  SenseConstraintTorque=off  SenseConstraintTorqueX=off  SenseConstraintTorqueY=off  SenseConstraintTorqueZ=off  SenseTotalForce=off  SenseTotalForceX=off  SenseTotalForceY=off  SenseTotalForceZ=off  SenseTotalTorque=off  SenseTotalTorqueX=off  SenseTotalTorqueY=off  SenseTotalTorqueZ=off  CompositeWrenchDir=FollowerOnBase  CompositeWrenchFrame=BaseFrame  EquilibriumPosition=0  EquilibriumPositionUnits=deg  SpringStiffness=0  SpringStiffnessUnits=N*m/deg  DampingCoefficient=0  DampingCoefficientUnits=N*m/(deg/s)  TorqueActuationMode=ComputedTorque  MotionActuationMode=InputMotion  SensePosition=on  SenseVelocity=off  SenseAcceleration=off  SenseTorqueForce=off  PositionTargetSpecify=off  PositionTargetPriority=High  PositionTargetValue=0  PositionTargetValueUnits=deg  VelocityTargetSpecify=off  VelocityTargetPriority=High  VelocityTargetValue=0  VelocityTargetValueUnits=deg/s  BlockFunction=simmechanics.library.joints.revolute_joint
  Rigid Transform : sm_lib/Frames and Transforms/Rigid Transform  TranslationMethod=StandardAxis  TranslationLengthUnit=m  TranslationStandardAxis=-X  TranslationStandardOffset=0.01  TranslationCartesianOffset=[0 0 0]  TranslationROffset=0  TranslationROffsetUnits=m  TranslationZOffset=0  TranslationZOffsetUnits=m  TranslationThetaOffset=0  TranslationThetaOffsetUnits=deg  RotationMethod=None  RotationAngleUnits=deg  RotationStandardAxis=+Z  RotationAngle=0.0  RotationArbitraryAxis=[0 0 1]  FollAlignAxisA=+X  BaseAlignAxisA=+Y  FollAlignAxisB=+Y  BaseAlignAxisB=+Z  RotationMatrix=[1 0 0; 0 1 0; 0 0 1]  BlockFunction=simmechanics.library.frames_transforms.rigid_transform
  Scope : Scope
      settings: YMin=0  YMax=14000  SaveName=ScopeData7
  Servo : Subsystem
  Servo1 : Subsystem
  Servo2 : Subsystem
  Simulink-PS Converter : nesl_utility/Simulink-PS Converter  PhysicalDomain=network_engine_domain  SubClassName=ps_input  LeftPortType=input  RightPortType=output  PseudoPeriodic=off  Frequencies=[]  NoiseDistribution=none  NoiseParameters=[]  Unit=1  AffineConversion=off  InputFiltering=on  SimscapeFilterOrder=2  InputFilterTimeConstant=0.001  UdotUserProvided=1
  Simulink-PS Converter1 : nesl_utility/Simulink-PS Converter  PhysicalDomain=network_engine_domain  SubClassName=ps_input  LeftPortType=input  RightPortType=output  PseudoPeriodic=off  Frequencies=[]  NoiseDistribution=none  NoiseParameters=[]  Unit=1  AffineConversion=off  InputFiltering=on  SimscapeFilterOrder=2  InputFilterTimeConstant=0.001  UdotUserProvided=1
  Simulink-PS Converter2 : nesl_utility/Simulink-PS Converter  PhysicalDomain=network_engine_domain  SubClassName=ps_input  LeftPortType=input  RightPortType=output  PseudoPeriodic=off  Frequencies=[]  NoiseDistribution=none  NoiseParameters=[]  Unit=1  AffineConversion=off  InputFiltering=on  SimscapeFilterOrder=2  InputFilterTimeConstant=0.001  UdotUserProvided=1
  Sphere to Plane Force : Contact_Forces_Lib/3D/Sphere to Plane Force  sphere_rad=0.01  plane_lenx=surfX  plane_leny=surfY  plane_depth=0.01/2  force_law=Linear  k_contact=23.9e3  b_contact=459  pen_full_damp_F=1e-4  pen_exponent=1  custom_param_1=1  custom_param_2=1  friction_law=Stick-Slip Continuous  mu_kinetic=2  mu_static=2  v_thr=0.001
  Sum : Sum  Inputs=|++
  Sum1 : Sum  Inputs=|+-
  Conn1 : PMIOPort  Port=1  Side=Left
  Conn2 : PMIOPort  Port=2  Side=Right
  Contact Force : Outport
  qReal : Outport  Port=2
  wires:
  Demux/2 -> Servo1/1(thetaRef)
  Demux/3 -> Servo2/1(thetaRef)
  Sum/1 -> Simulink-PS Converter2/1
  Constant3/1 -> Sum/2
  Demux/1 -> Servo/1(thetaRef)
  qRef/1 -> Demux/1
  Servo/1(theta) -> Simulink-PS Converter/1
  Servo1/1(theta) -> Simulink-PS Converter1/1
  Servo2/1(theta) -> Sum/1
  Sphere to Plane Force/1 -> Bus Selector/1
  Bus Selector/1 -> Contact Force/1, Scope/1  "<Normal Force>"
  Mux/1 -> qReal/1
  PS-Simulink Converter2/1 -> Mux/1
  PS-Simulink Converter1/1 -> Mux/2
  PS-Simulink Converter/1 -> Sum1/1
  Sum1/1 -> Mux/3
  Constant1/1 -> Sum1/2
  connections:
  Link1/LConn1 -- Revolute Joint/RConn1
  Revolute Joint/LConn1 -- Conn1/RConn1
  Revolute Joint/LConn2 -- Simulink-PS Converter/RConn1
  Revolute Joint1/LConn1 -- Link1/RConn1
  Revolute Joint1/RConn1 -- Link2/LConn1
  Revolute Joint2/LConn1 -- Link2/RConn1
  Revolute Joint2/RConn1 -- Link3/LConn1
  Simulink-PS Converter1/RConn1 -- Revolute Joint1/LConn2
  Revolute Joint2/LConn2 -- Simulink-PS Converter2/RConn1
  Rigid Transform/LConn1 -- Link3/RConn1
  Sphere to Plane Force/RConn1 -- Conn2/RConn1
  PS-Simulink Converter/LConn1 -- Revolute Joint2/RConn2
  PS-Simulink Converter1/LConn1 -- Revolute Joint1/RConn2
  PS-Simulink Converter2/LConn1 -- Revolute Joint/RConn2
  Sphere to Plane Force/LConn1 -- Rigid Transform/RConn1
